simulink model "EJ3_2_1_Simulink"  (R2014a)
settings: Solver=ode45  StartTime=0.0  StopTime=10.0  RelTol=1e-3
values from neighbouring files (symbols this model uses):
  den = den'    [EJ4_1.m]
undefined symbols (not defined in the file or in its folder): den1, den2, den22, den3, num, num1, num2, num22, num3
settings Model: Creator=lraff  LastModifiedBy=lraff

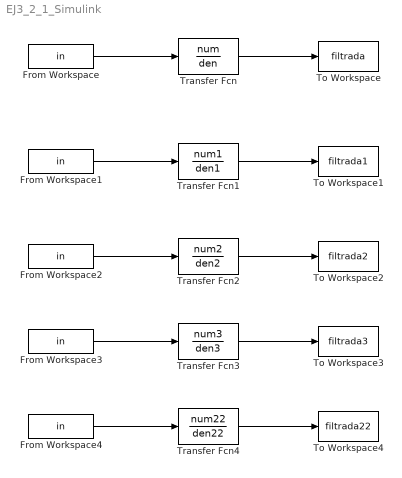
== system EJ3_2_1_Simulink ==
  From Workspace{,1..4} (5 alike) : FromWorkspace  VariableName=in  SampleTime=0
  To Workspace : ToWorkspace  VariableName=filtrada  SaveFormat=Structure With Time  SampleTime=9.07e-5
  To Workspace1 : ToWorkspace  VariableName=filtrada1  SaveFormat=Structure With Time  SampleTime=9.07e-5
  To Workspace2 : ToWorkspace  VariableName=filtrada2  SaveFormat=Structure With Time  SampleTime=9.07e-5
  To Workspace3 : ToWorkspace  VariableName=filtrada3  SaveFormat=Structure With Time  SampleTime=9.07e-5
  To Workspace4 : ToWorkspace  VariableName=filtrada22  SaveFormat=Structure With Time  SampleTime=9.07e-5
  Transfer Fcn : TransferFcn  Numerator=num  Denominator=den
  Transfer Fcn1 : TransferFcn  Numerator=num1  Denominator=den1
  Transfer Fcn2 : TransferFcn  Numerator=num2  Denominator=den2
  Transfer Fcn3 : TransferFcn  Numerator=num3  Denominator=den3
  Transfer Fcn4 : TransferFcn  Numerator=num22  Denominator=den22
  wires:
  From Workspace/1 -> Transfer Fcn/1
  Transfer Fcn/1 -> To Workspace/1
  From Workspace1/1 -> Transfer Fcn1/1
  Transfer Fcn1/1 -> To Workspace1/1
  From Workspace2/1 -> Transfer Fcn2/1
  Transfer Fcn2/1 -> To Workspace2/1
  From Workspace3/1 -> Transfer Fcn3/1
  Transfer Fcn3/1 -> To Workspace3/1
  From Workspace4/1 -> Transfer Fcn4/1
  Transfer Fcn4/1 -> To Workspace4/1
